simulink model "l_ctrl"  (R2023b)
settings: configuration reference "ctrl_tsk_conf" (kept outside this file)
settings Model: DataDictionary=fmuGenerationDictionay.sldd  ModifiedByFormat=Third Equation Ltd  Creator=Third Equation Ltd  LastModifiedBy=Third Equation Ltd
settings ConfigSetRef: SourceName=ctrl_tsk_conf

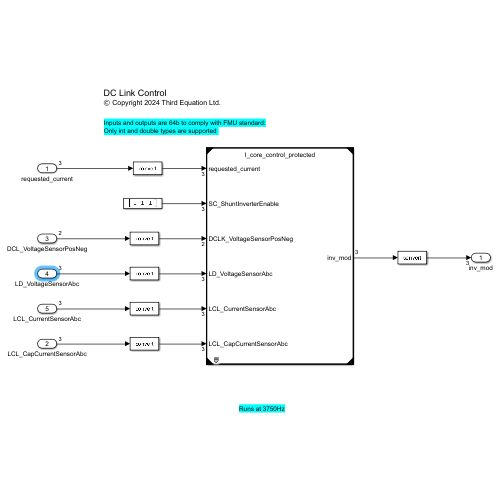
[thumbnail: Simulink's stored preview of the top-level diagram]
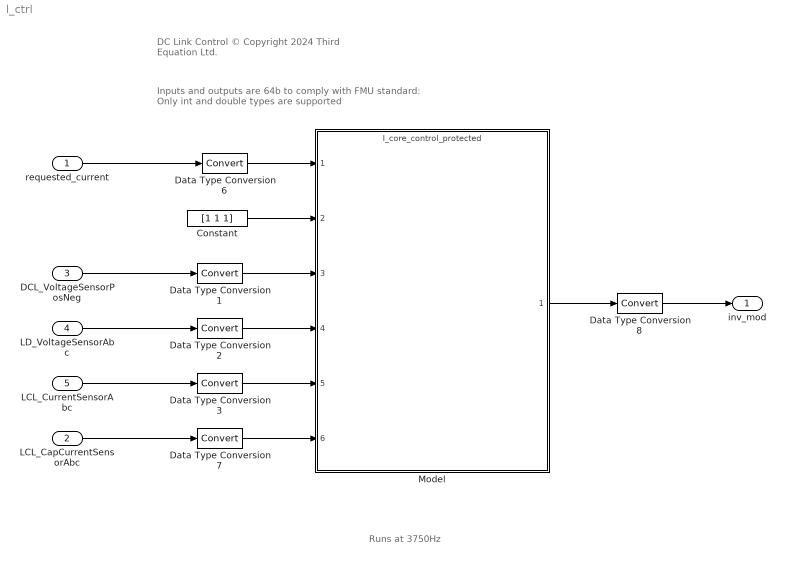
== system l_ctrl ==
  note: Inputs and outputs are 64b to comply with FMU standard:
      | Only int and double types are supported
  note: DC Link Control
      | © Copyright 2024 Third Equation Ltd.
  note: Runs at 3750Hz
  requested_current : Inport  OutDataTypeStr=double  PortDimensions=3
  LCL_CapCurrentSensorAbc : Inport  Port=2  OutDataTypeStr=double  PortDimensions=3
  DCL_VoltageSensorPosNeg : Inport  Port=3  OutDataTypeStr=double  PortDimensions=2
  LD_VoltageSensorAbc : Inport  Port=4  OutDataTypeStr=double  PortDimensions=3
  LCL_CurrentSensorAbc : Inport  Port=5  OutDataTypeStr=double  PortDimensions=3
  Constant : Constant  Value=[1 1 1]  OutDataTypeStr=boolean
  Data Type Conversion{1..3,6..8} (6 alike) : DataTypeConversion  SaturateOnIntegerOverflow=off  RndMeth=Floor
  Model : ModelReference  ModelNameDialog=I_core_control_protected.slxp  ModelReferenceVersion=1.28  CopyOfModelProtected=on
  inv_mod : Outport  OutDataTypeStr=double  PortDimensions=3
  wires:
  Data Type Conversion6/1 -> Model/1
  requested_current/1 -> Data Type Conversion6/1
  LCL_CapCurrentSensorAbc/1 -> Data Type Conversion7/1
  Model/1 -> Data Type Conversion8/1
  Data Type Conversion8/1 -> inv_mod/1
  Constant/1 -> Model/2
  Data Type Conversion7/1 -> Model/6
  Data Type Conversion3/1 -> Model/5
  Data Type Conversion2/1 -> Model/4
  Data Type Conversion1/1 -> Model/3
  DCL_VoltageSensorPosNeg/1 -> Data Type Conversion1/1
  LD_VoltageSensorAbc/1 -> Data Type Conversion2/1
  LCL_CurrentSensorAbc/1 -> Data Type Conversion3/1
